simulink model "Model"  (R2020b)
settings: Solver=FixedStepDiscrete  StartTime=0.0  StopTime=10  FixedStep=0.1  RelTol=1e-3
settings Model: Creator=FM5  LastModifiedBy=FM5

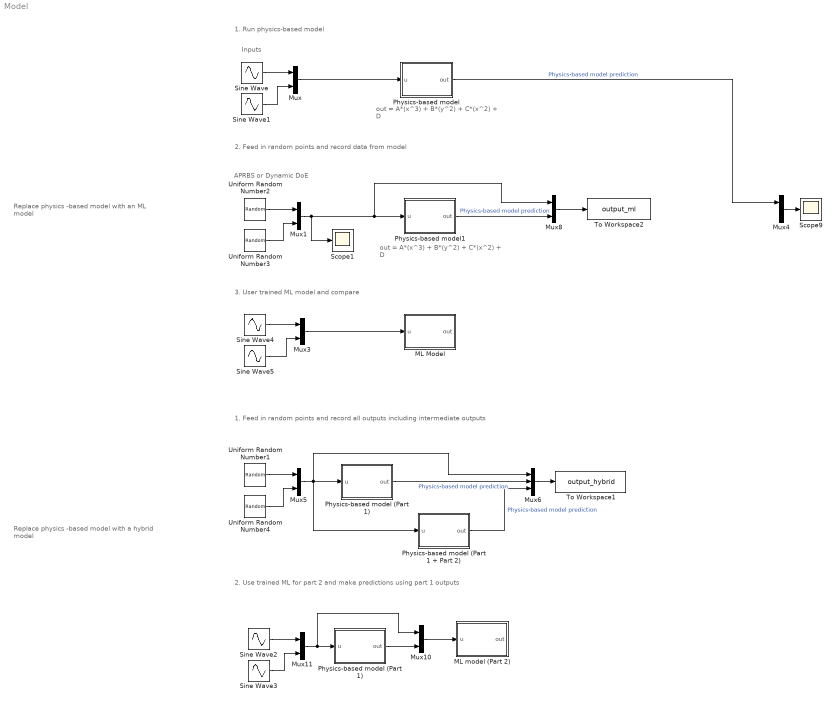
== system Model ==
  note: out = A*(x^3) + B*(y^2) + C*(x^2) + D
  note: Inputs
  note: APRBS or
      | Dynamic DoE
  note: out = A*(x^3) + B*(y^2) + C*(x^2) + D
  note: 1. Run physics-based model
  note: 2. Feed in random points and record data from model
  note: 3. User trained ML model and compare
  note: Replace physics -based model with an ML model
  note: Replace physics -based model with a hybrid model
  note: 1. Feed in random points and record all outputs including intermediate outputs
  note: 2. Use trained ML for part 2 and make predictions using part 1 outputs
  ML Model : MATLAB Function  TreatAsAtomicUnit=on
  "ML model (Part 2) " : MATLAB Function  TreatAsAtomicUnit=on
  Mux{,1,3,5,8,10..11} (7 alike) : Mux  Inputs=2
  Mux4 : Mux  Inputs=3
  Mux6 : Mux  Inputs=3
  Physics-based model : MATLAB Function  TreatAsAtomicUnit=on
  Physics-based model (Part 1 + Part 2) : MATLAB Function  TreatAsAtomicUnit=on
  Physics-based model (Part 1) : MATLAB Function  TreatAsAtomicUnit=on
  "Physics-based model (Part 1) " : MATLAB Function  TreatAsAtomicUnit=on
  Physics-based model1 : MATLAB Function  TreatAsAtomicUnit=on
  Scope1 : Scope
  Scope9 : Scope
  Sine Wave : Sin  Bias=1  SampleTime=0
  Sine Wave1 : Sin  Bias=1  Phase=12  SampleTime=0
  Sine Wave2 : Sin  Bias=1  SampleTime=0
  Sine Wave3 : Sin  Bias=1  Phase=12  SampleTime=0
  Sine Wave4 : Sin  Bias=1  SampleTime=0
  Sine Wave5 : Sin  Bias=1  Phase=12  SampleTime=0
  To Workspace1 : ToWorkspace  VariableName=output_hybrid  SampleTime=-1
      settings: Save2DSignal=2-D array (concatenate along first dimension)
  To Workspace2 : ToWorkspace  VariableName=output_ml  SampleTime=-1
      settings: Save2DSignal=2-D array (concatenate along first dimension)
  Uniform Random Number1 : UniformRandomNumber  Minimum=0  Maximum=2  SampleTime=0.1
  Uniform Random Number2 : UniformRandomNumber  Minimum=0  Maximum=2  SampleTime=0.1
  Uniform Random Number3 : UniformRandomNumber  Minimum=0  Maximum=2  Seed=1  SampleTime=0.1
  Uniform Random Number4 : UniformRandomNumber  Minimum=0  Maximum=2  Seed=1  SampleTime=0.1
  wires:
  Sine Wave1/1 -> Mux/2
  Sine Wave/1 -> Mux/1
  Physics-based model/1(out) -> Mux4/1  "Physics-based model prediction"
  Uniform Random Number3/1 -> Mux1/2
  Uniform Random Number2/1 -> Mux1/1
  Sine Wave4/1 -> Mux3/1
  Mux3/1 -> ML Model/1(u)
  Sine Wave5/1 -> Mux3/2
  Mux4/1 -> Scope9/1
  Mux6/1 -> To Workspace1/1
  Uniform Random Number1/1 -> Mux5/1
  Uniform Random Number4/1 -> Mux5/2
  Mux/1 -> Physics-based model/1(u)
  Mux5/1 -> Mux6/1, Physics-based model (Part 1 + Part 2)/1(u), Physics-based model (Part 1)/1(u)
  Physics-based model (Part 1)/1(out) -> Mux6/2  "Physics-based model prediction"
  Mux10/1 -> "ML model (Part 2) "/1(u)
  Mux11/1 -> Mux10/1, "Physics-based model (Part 1) "/1(u)
  "Physics-based model (Part 1) "/1(out) -> Mux10/2
  Sine Wave3/1 -> Mux11/2
  Sine Wave2/1 -> Mux11/1
  Mux1/1 -> Mux8/1, Physics-based model1/1(u), Scope1/1
  Physics-based model1/1(out) -> Mux8/2  "Physics-based model prediction"
  Mux8/1 -> To Workspace2/1
  Physics-based model (Part 1 + Part 2)/1(out) -> Mux6/3  "Physics-based model prediction"

== matlab function Model/Physics-based model ==
  data: u input; out output


function out = fcn(u)

x = u(1);
y = u(2);

A = 2;
B = 1;
C = 3;
D = 2;

out = A*(x^3) + B*(y^2) + C*(x^2) + D;

== matlab function Model/ML Model ==
  data: u input; out output
function out = fcn(u)

% Initialise
out = 1;

% Declare predict as extrinsic function
coder.extrinsic('predict')
coder.extrinsic('loadCompactModel')

% Load ML model
mdl = loadCompactModel('TrainedModel');

% Run prediction
out = predict(mdl,[u(1) u(2)]);

== matlab function Model/Physics-based model1 ==
  data: u input; out output
function out = fcn(u)

x = u(1);
y = u(2);

A = 2;
B = 1;
C = 3;
D = 2;

out = A*(x^3) + B*(y^2) + C*(x^2) + D;

== matlab function Model/Physics-based model (Part 1) ==
  data: u input; out output
function out = fcn(u)

x = u(1);
y = u(2);

A = 2;
B = 1;

out = A*(x^3) + B*(y^2);

== matlab function Model/ML model (Part 2)  ==
  data: u input; out output
function out = fcn(u)

% Initialise
out = 1;

% Declare predict as extrinsic function
coder.extrinsic('predict')
coder.extrinsic('loadCompactModel')

% Load ML model
mdl = loadCompactModel('TrainedModel_hybrid');

% Run prediction
out = predict(mdl,[u(1) u(2) u(3)]);

== matlab function Model/Physics-based model (Part 1)  ==
  data: u input; out output
function out = fcn(u)

x = u(1);
y = u(2);

A = 2;
B = 1;

out = A*(x^3) + B*(y^2);

== matlab function Model/Physics-based model (Part 1 + Part 2) ==
  data: u input; out output
function out = fcn(u)

x = u(1);
y = u(2);

A = 2;
B = 1;
C = 3;
D = 2;

Part1 = A*(x^3) + B*(y^2);
Part2 = C*(x^2) + D;

out = Part1 + Part2;
